simulink model "LQR"  (R2017a)
settings: Solver=FixedStepAuto  StartTime=0.0  StopTime=10  FixedStep=0.0001  RelTol=1e-3
values from neighbouring files (symbols this model uses):
  As = [-(2*Cf+2*Cr)/(m*Vx) (-lf*2*Cf+lr*2*Cr)/(m*Vx)-Vx 0 ... (first row only)    [LQR_Setup_2017.m]
  Bs = [Cf/m, (2*Cf*lf)/Iz 0]'    [LQR_Setup_2017.m]
  K1 = K(1,1)    [LQR_Setup_2017.m]
  K2 = K(1,2)    [LQR_Setup_2017.m]
  K3 = K(1,3)    [LQR_Setup_2017.m]
undefined symbols (not defined in the file or in its folder): DiscIntNeverNeededParam
settings Model: Creator=Johan PC  LastModifiedBy=Johan PC
settings SFSimCC: SimUseLocalCustomCode=on
settings RTWCC: RTWUseLocalCustomCode=on

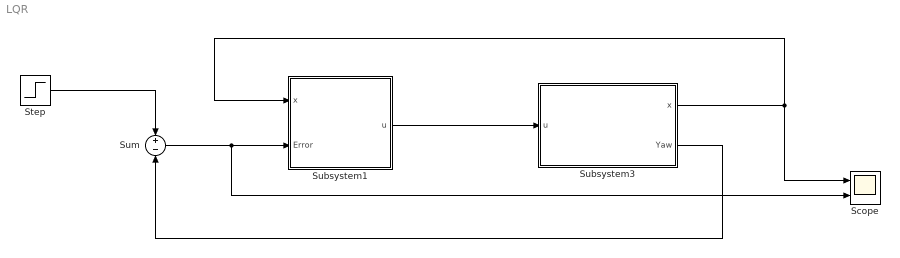
== system LQR ==
  Scope : Scope  NumInputPorts=2
  Step : Step  Time=0.5  SampleTime=0
  Subsystem1 : Subsystem
  Subsystem3 : Subsystem
  Sum : Sum  Inputs=+-
  wires:
  Sum/1 -> Scope/2, Subsystem1/2(Error)
  Subsystem3/1(x) -> Subsystem1/1(x), Scope/1
  Subsystem3/2(Yaw) -> Sum/2
  Subsystem1/1(u) -> Subsystem3/1(u)
  Step/1 -> Sum/1

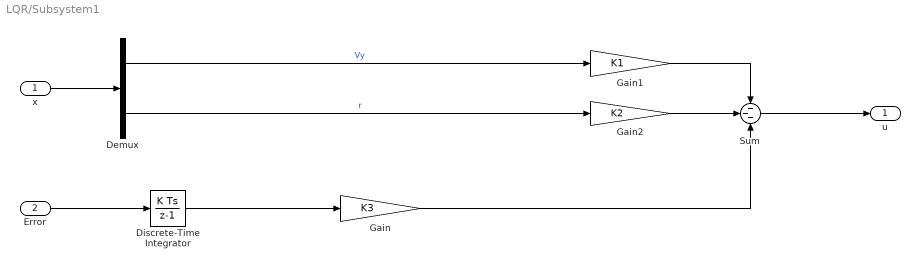
== system LQR/Subsystem1 ==
  x : Inport
  Error : Inport  Port=2
  Demux : Demux  Outputs=2
  Discrete-Time Integrator : DiscreteIntegrator  InitialConditionSetting=State (most efficient)  SampleTime=0.001  ICPrevOutput=DiscIntNeverNeededParam  ICPrevScaledInput=DiscIntNeverNeededParam
  Gain : Gain  Gain=K3
  Gain1 : Gain  Gain=K1
  Gain2 : Gain  Gain=K2
  Sum : Sum  Inputs=---
  u : Outport
  wires:
  Error/1 -> Discrete-Time Integrator/1
  Discrete-Time Integrator/1 -> Gain/1
  Gain/1 -> Sum/3
  x/1 -> Demux/1
  Demux/1 -> Gain1/1  "Vy"
  Demux/2 -> Gain2/1  "r"
  Gain1/1 -> Sum/1
  Gain2/1 -> Sum/2
  Sum/1 -> u/1

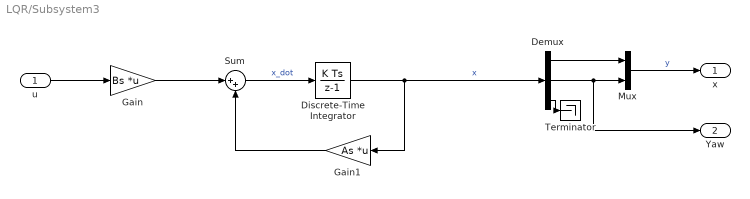
== system LQR/Subsystem3 ==
  u : Inport
  Demux : Demux  Outputs=3
  Discrete-Time Integrator : DiscreteIntegrator  InitialConditionSetting=State (most efficient)  SampleTime=0.0001  ICPrevOutput=DiscIntNeverNeededParam  ICPrevScaledInput=DiscIntNeverNeededParam
  Gain : Gain  Gain=Bs  Multiplication=Matrix(K*u)
  Gain1 : Gain  Gain=As  Multiplication=Matrix(K*u)
  Mux : Mux  Inputs=2
  Sum : Sum  Inputs=|++
  Terminator : Terminator
  x : Outport
  Yaw : Outport  Port=2
  wires:
  Discrete-Time Integrator/1 -> Gain1/1, Demux/1  "x"
  Gain1/1 -> Sum/2
  Gain/1 -> Sum/1
  Sum/1 -> Discrete-Time Integrator/1  "x_dot"
  u/1 -> Gain/1
  Mux/1 -> x/1  "y"
  Demux/2 -> Yaw/1, Mux/2
  Demux/1 -> Mux/1
  Demux/3 -> Terminator/1
